simulink model "MARS1"  (R2022a)
settings: Solver=VariableStepAuto  StartTime=0.0  StopTime=inf  RelTol=1e-3
InitFcn:
  | links = gzlink("list","ingenuity");
  | for i=1:length(links)
  | gzlink("set","ingenuity",links(i),"Gravity","off");
  | end
model workspace (MAT data in the model file):
  T0 = -23.4
  h_trop = 7
  ingenuityParams : object (value not decoded)
values from neighbouring files (symbols this model uses):
  ingenuityParams =     [marsBatParam.mat]
undefined symbols (not defined in the file or in its folder): body, collective1, collective2, duration, ingenuity, leg1, leg2, leg3, leg4, link_name, model_name, rotor1, rotor2, solarPanel, world_pose
libraries: fl_lib x35, robotgazebolib x31, nesl_utility x12, ee_lib x11, slpidlib x7, simulink x4, sharedtransform x2, shared6dof x1, aerolibwind2 x1
(part 2 of 3)

== system MARS1/Gazebo Simulation/Link Body6 ==
  In1 : Inport
  In2 : Inport  Port=2
  In3 : Inport  Port=3
  In4 : Inport  Port=4
  In5 : Inport  Port=5
  In6 : Inport  Port=6
  In7 : Inport  Port=7
  In8 : Inport  Port=8
  Bus Assignment : BusAssignment  AssignedSignals=model_name,link_name,world_pose.position.x,world_pose.position.y,world_pose.position.z,world_pose.orientation.w,world_pose.orientation.x,world_pose.orientation.y,world_pose.orientation.z,duration.seconds
  Gazebo Blank Message : robotgazebolib/Gazebo Blank Message  msgType=SetLinkWorldPose  sampleTime=0.01  busName='Gazebo_SL_Bus_gazebo_msgs_SetLinkWorldPose'
      settings: SourceProductBaseCode=RO
  Gazebo Select Entity : robotgazebolib/Gazebo Select Entity  modelElemName=ingenuity/collective1  outputArraySize=128  OutputLabel=Link  SelectType=Link
      settings: SourceProductBaseCode=RO
  Out1 : Outport
  wires:
  In6/1 -> Bus Assignment/9
  In4/1 -> Bus Assignment/7
  In3/1 -> Bus Assignment/6
  In7/1 -> Bus Assignment/10
  In2/1 -> Bus Assignment/5
  Bus Assignment/1 -> Out1/1
  Gazebo Select Entity/2 -> Bus Assignment/3
  In5/1 -> Bus Assignment/8
  Gazebo Blank Message/1 -> Bus Assignment/1
  In8/1 -> Bus Assignment/11
  In1/1 -> Bus Assignment/4
  Gazebo Select Entity/1 -> Bus Assignment/2

== system MARS1/Gazebo Simulation/Link Body7 ==
  In1 : Inport
  In2 : Inport  Port=2
  In3 : Inport  Port=3
  In4 : Inport  Port=4
  In5 : Inport  Port=5
  In6 : Inport  Port=6
  In7 : Inport  Port=7
  In8 : Inport  Port=8
  Bus Assignment : BusAssignment  AssignedSignals=model_name,link_name,world_pose.position.x,world_pose.position.y,world_pose.position.z,world_pose.orientation.w,world_pose.orientation.x,world_pose.orientation.y,world_pose.orientation.z,duration.seconds
  Gazebo Blank Message : robotgazebolib/Gazebo Blank Message  msgType=SetLinkWorldPose  sampleTime=0.01  busName='Gazebo_SL_Bus_gazebo_msgs_SetLinkWorldPose'
      settings: SourceProductBaseCode=RO
  Gazebo Select Entity : robotgazebolib/Gazebo Select Entity  modelElemName=ingenuity/rotor1  outputArraySize=128  OutputLabel=Link  SelectType=Link
      settings: SourceProductBaseCode=RO
  Out1 : Outport
  wires:
  Gazebo Select Entity/1 -> Bus Assignment/2
  In1/1 -> Bus Assignment/4
  In8/1 -> Bus Assignment/11
  Gazebo Blank Message/1 -> Bus Assignment/1
  In5/1 -> Bus Assignment/8
  Gazebo Select Entity/2 -> Bus Assignment/3
  Bus Assignment/1 -> Out1/1
  In2/1 -> Bus Assignment/5
  In7/1 -> Bus Assignment/10
  In3/1 -> Bus Assignment/6
  In4/1 -> Bus Assignment/7
  In6/1 -> Bus Assignment/9

== system MARS1/Gazebo Simulation/Link Body8 ==
  In1 : Inport
  In2 : Inport  Port=2
  In3 : Inport  Port=3
  In4 : Inport  Port=4
  In5 : Inport  Port=5
  In6 : Inport  Port=6
  In7 : Inport  Port=7
  In8 : Inport  Port=8
  Bus Assignment : BusAssignment  AssignedSignals=model_name,link_name,world_pose.position.x,world_pose.position.y,world_pose.position.z,world_pose.orientation.w,world_pose.orientation.x,world_pose.orientation.y,world_pose.orientation.z,duration.seconds
  Gazebo Blank Message : robotgazebolib/Gazebo Blank Message  msgType=SetLinkWorldPose  sampleTime=0.01  busName='Gazebo_SL_Bus_gazebo_msgs_SetLinkWorldPose'
      settings: SourceProductBaseCode=RO
  Gazebo Select Entity : robotgazebolib/Gazebo Select Entity  modelElemName=ingenuity/body  outputArraySize=128  OutputLabel=Link  SelectType=Link
      settings: SourceProductBaseCode=RO
  Out1 : Outport
  wires:
  In6/1 -> Bus Assignment/9
  In4/1 -> Bus Assignment/7
  In3/1 -> Bus Assignment/6
  In7/1 -> Bus Assignment/10
  In2/1 -> Bus Assignment/5
  Bus Assignment/1 -> Out1/1
  Gazebo Select Entity/2 -> Bus Assignment/3
  In5/1 -> Bus Assignment/8
  Gazebo Blank Message/1 -> Bus Assignment/1
  In8/1 -> Bus Assignment/11
  In1/1 -> Bus Assignment/4
  Gazebo Select Entity/1 -> Bus Assignment/2

== system MARS1/Gazebo Simulation/Link Body9 ==
  In1 : Inport
  In2 : Inport  Port=2
  In3 : Inport  Port=3
  In4 : Inport  Port=4
  In5 : Inport  Port=5
  In6 : Inport  Port=6
  In7 : Inport  Port=7
  In8 : Inport  Port=8
  Bus Assignment : BusAssignment  AssignedSignals=model_name,link_name,world_pose.position.x,world_pose.position.y,world_pose.position.z,world_pose.orientation.w,world_pose.orientation.x,world_pose.orientation.y,world_pose.orientation.z,duration.seconds
  Gazebo Blank Message : robotgazebolib/Gazebo Blank Message  msgType=SetLinkWorldPose  sampleTime=0.01  busName='Gazebo_SL_Bus_gazebo_msgs_SetLinkWorldPose'
      settings: SourceProductBaseCode=RO
  Gazebo Select Entity : robotgazebolib/Gazebo Select Entity  modelElemName=ingenuity/leg4  outputArraySize=128  OutputLabel=Link  SelectType=Link
      settings: SourceProductBaseCode=RO
  Out1 : Outport
  wires:
  Gazebo Select Entity/1 -> Bus Assignment/2
  In1/1 -> Bus Assignment/4
  In8/1 -> Bus Assignment/11
  Gazebo Blank Message/1 -> Bus Assignment/1
  In5/1 -> Bus Assignment/8
  Gazebo Select Entity/2 -> Bus Assignment/3
  Bus Assignment/1 -> Out1/1
  In2/1 -> Bus Assignment/5
  In7/1 -> Bus Assignment/10
  In3/1 -> Bus Assignment/6
  In4/1 -> Bus Assignment/7
  In6/1 -> Bus Assignment/9

== system MARS1/Gazebo Simulation/Rot2Quat ==
  "R1, R2, R3" : Inport
  Demux : Demux
  Rate w : RateTransition
  Rate x : RateTransition
  Rate y : RateTransition
  Rate z : RateTransition
  Rotation Angles to Quaternions : sharedtransform/Rotation Angles to Quaternions  rotationOrder=XYZ  aMode=aMode
      settings: SourceProductBaseCode=AE,PW,DR,MT,VE
  Out1 : Outport
  Out2 : Outport  Port=2
  Out3 : Outport  Port=3
  Out4 : Outport  Port=4
  wires:
  Demux/3 -> Rate y/1
  Demux/2 -> Rate x/1
  Demux/1 -> Rate w/1
  Demux/4 -> Rate z/1
  Rate x/1 -> Out2/1
  Rotation Angles to Quaternions/1 -> Demux/1
  "R1, R2, R3"/1 -> Rotation Angles to Quaternions/1
  Rate y/1 -> Out3/1
  Rate w/1 -> Out1/1
  Rate z/1 -> Out4/1

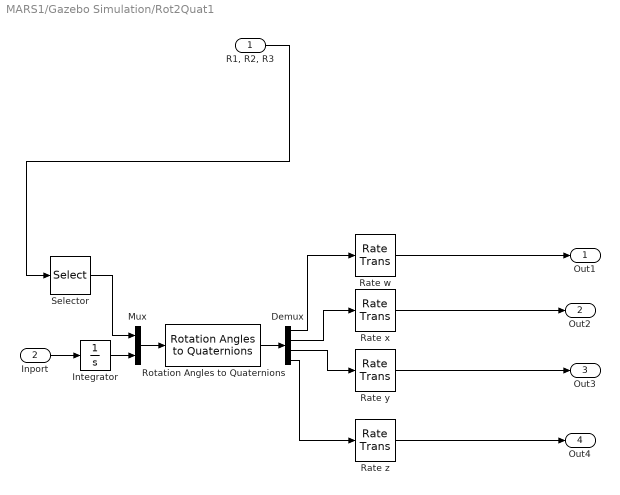
== system MARS1/Gazebo Simulation/Rot2Quat1 ==
  "R1, R2, R3" : Inport
  Inport : Inport  Port=2
  Demux : Demux
  Integrator : Integrator
  Mux : Mux  Inputs=2
  Rate w : RateTransition
  Rate x : RateTransition
  Rate y : RateTransition
  Rate z : RateTransition
  Rotation Angles to Quaternions : sharedtransform/Rotation Angles to Quaternions  rotationOrder=XYZ  aMode=aMode
      settings: SourceProductBaseCode=AE,PW,DR,MT,VE
  Selector : Selector  InputPortWidth=3  IndexOptions=Index vector (dialog)  Indices=[1 2]  OutputSizes=1
  Out1 : Outport
  Out2 : Outport  Port=2
  Out3 : Outport  Port=3
  Out4 : Outport  Port=4
  wires:
  Rate z/1 -> Out4/1
  Rate w/1 -> Out1/1
  Rate y/1 -> Out3/1
  Rotation Angles to Quaternions/1 -> Demux/1
  Rate x/1 -> Out2/1
  Demux/4 -> Rate z/1
  Demux/1 -> Rate w/1
  Demux/2 -> Rate x/1
  Demux/3 -> Rate y/1
  Mux/1 -> Rotation Angles to Quaternions/1
  Selector/1 -> Mux/1
  "R1, R2, R3"/1 -> Selector/1
  Integrator/1 -> Mux/2
  Inport/1 -> Integrator/1

== system MARS1/Gazebo Simulation/xyz ==
  In1 : Inport
  Demux1 : Demux  Outputs=3
  Rate Transition : RateTransition
  Rate Transition1 : RateTransition
  Rate Transition2 : RateTransition
  Out1 : Outport
  Out2 : Outport  Port=2
  Out3 : Outport  Port=3
  wires:
  Demux1/3 -> Rate Transition2/1
  Demux1/1 -> Rate Transition/1
  Demux1/2 -> Rate Transition1/1
  In1/1 -> Demux1/1
  Rate Transition/1 -> Out1/1
  Rate Transition1/1 -> Out2/1
  Rate Transition2/1 -> Out3/1

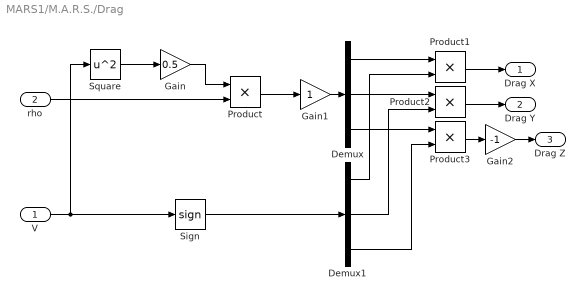
== system MARS1/M.A.R.S./Drag ==
  V : Inport
  rho : Inport  Port=2
  Demux : Demux  Outputs=3
  Demux1 : Demux  Outputs=3
  Gain : Gain  Gain=0.5
  Gain1 : Gain
  Gain2 : Gain  Gain=-1
  Product{,1..3} (4 alike) : Product
  Sign : Signum
  Square : Math  Operator=square
  Drag X : Outport
  Drag Y : Outport  Port=2
  Drag Z : Outport  Port=3
  wires:
  V/1 -> Square/1, Sign/1
  Demux1/3 -> Product3/2
  Demux1/2 -> Product2/2
  Demux/3 -> Product3/1
  Gain/1 -> Product/1
  Gain1/1 -> Demux/1
  rho/1 -> Product/2
  Square/1 -> Gain/1
  Demux1/1 -> Product1/2
  Product/1 -> Gain1/1
  Product1/1 -> Drag X/1
  Demux/1 -> Product1/1
  Demux/2 -> Product2/1
  Sign/1 -> Demux1/1
  Product2/1 -> Drag Y/1
  Product3/1 -> Gain2/1
  Gain2/1 -> Drag Z/1

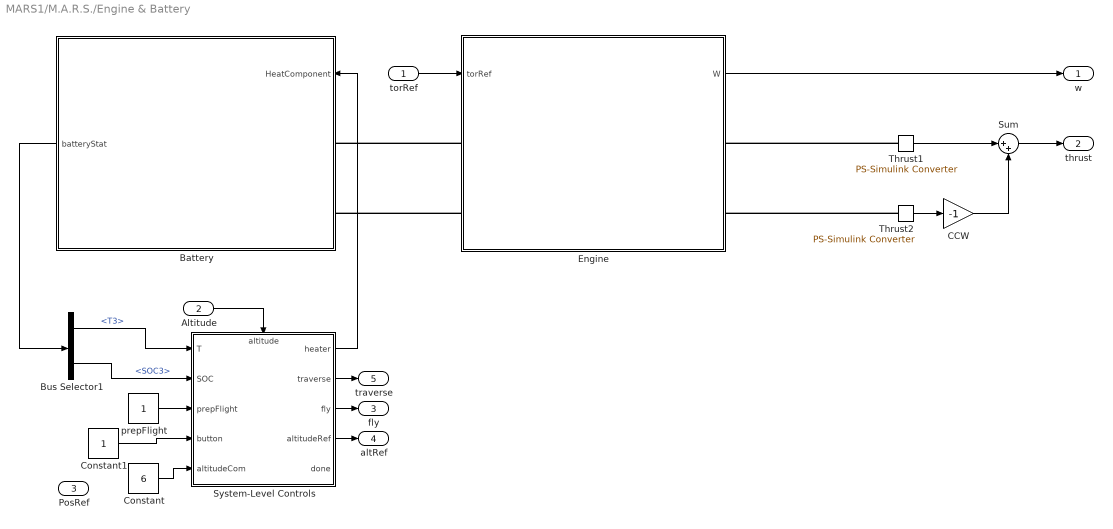
== system MARS1/M.A.R.S./Engine & Battery ==
  torRef : Inport
  Altitude : Inport  Port=2
  PosRef : Inport  Port=3
  Battery : Subsystem
      mask Display: image('$imagefile'); % Use "Edit Image" on toolstrip to change.
  Bus Selector1 : BusSelector  OutputSignals=T3,SOC3
  CCW : Gain  Gain=-1
  Constant : Constant  Value=6
  Constant1 : Constant
  Engine : Subsystem
      mask Display: image('$imagefile'); % Use "Edit Image" on toolstrip to change.
  Sum : Sum  Inputs=|++
  System-Level Controls : Stateflow chart  TreatAsAtomicUnit=on
      settings: PortSchema="{\"entries\":[{\"content\":{\"sides\":[{\"content\":{\"connectorIds\":[\"In2\",\"In3\",\"In5\",\"In4\",\"In1\"]},\"type\":\"ConnectorPlacement.EquallySpacedRectSide\",\"uuid\":\"5067341e-d12a-4a2a-9253-3fb06d0079cf\"},{\"content\":{\"connectorIds\":[\"Out1\",\"Out2\",\"Out3\",\"Out4\",\"Out5\"],\"side\":\"RIGHT\"},\"type\":\"ConnectorPlacement.EquallySpacedRectSide\",\"uuid\":\"5404e1d9-f923-45fb-998d-e24e5a5fd6b6\"},{\"content\":{\"connectorIds\":[\"In6\"],\"side\":\"TOP\"},\"type\":\"ConnectorPlacement.EquallySpacedRectSide\",\"uuid\":\"b72b8578-46c7-4b5e-a689-fe24a80a6d63\"}]},\"type\":\"ConnectorPlacement.EquallySpacedConnector\",\"uuid\":\"f5827d07-5d2a-4259-8e8b-6d4ada56c462\"}],\"packageUris\":[\"http://schema.mathworks.com/mf0/Connector/R2020b\"],\"version\":\"1.0\"}"
  Thrust1 : nesl_utility/PS-Simulink Converter  PhysicalDomain=network_engine_domain  SubClassName=ps_output  LeftPortType=input  RightPortType=output  PseudoPeriodic=off  Frequencies=[]  VectorFormat=inherit  Unit=inherit  AffineConversion=off
      settings: SourceProductBaseCode=SS,PW,VE
  Thrust2 : nesl_utility/PS-Simulink Converter  PhysicalDomain=network_engine_domain  SubClassName=ps_output  LeftPortType=input  RightPortType=output  PseudoPeriodic=off  Frequencies=[]  VectorFormat=inherit  Unit=inherit  AffineConversion=off
      settings: SourceProductBaseCode=SS,PW,VE
  prepFlight : Constant
  w : Outport
  thrust : Outport  Port=2
  fly : Outport  Port=3
  altRef : Outport  Port=4
  traverse : Outport  Port=5
  wires:
  Thrust2/1 -> CCW/1
  Sum/1 -> thrust/1
  System-Level Controls/1(heater) -> Battery/1(HeatComponent)
  Battery/1(batteryStat) -> Bus Selector1/1
  System-Level Controls/3(fly) -> fly/1
  Bus Selector1/2 -> System-Level Controls/3(SOC)  "<SOC3>"
  Bus Selector1/1 -> System-Level Controls/2(T)  "<T3>"
  System-Level Controls/4(altitudeRef) -> altRef/1
  prepFlight/1 -> System-Level Controls/5(prepFlight)
  Altitude/1 -> System-Level Controls/6(altitude)
  Constant/1 -> System-Level Controls/1(altitudeCom)
  Thrust1/1 -> Sum/1
  CCW/1 -> Sum/2
  torRef/1 -> Engine/1(torRef)
  Engine/1(W) -> w/1
  System-Level Controls/2(traverse) -> traverse/1
  Constant1/1 -> System-Level Controls/4(button)
  connections:
  Thrust1/LConn1 -- Engine/RConn1
  Engine/LConn1 -- Battery/LConn1
  Engine/LConn2 -- Battery/LConn2
  Thrust2/LConn1 -- Engine/RConn2

== system MARS1/M.A.R.S./Force Components ==
  note: Subsystem
  In1 : Inport
  In2 : Inport  Port=2
  delta : Inport  Port=3
  epsilon : Inport  Port=4
  Components : Subsystem
  Product2 : Product
  Subsystem : Subsystem
  Out1 : Outport
  Out2 : Outport  Port=2
  Out3 : Outport  Port=3
  wires:
  Components/2(Out2) -> Subsystem/3(In3)
  Components/1(Out1) -> Subsystem/2(In2)
  Components/3(Out3) -> Subsystem/4(In4)
  In1/1 -> Product2/1
  Components/4(Out4) -> Subsystem/5(In5)
  epsilon/1 -> Components/2(epsilon)
  Subsystem/1(Out1) -> Out1/1
  Product2/1 -> Subsystem/1(In1)
  delta/1 -> Components/1(delta)
  In2/1 -> Product2/2
  Subsystem/3(Out3) -> Out3/1
  Subsystem/2(Out2) -> Out2/1

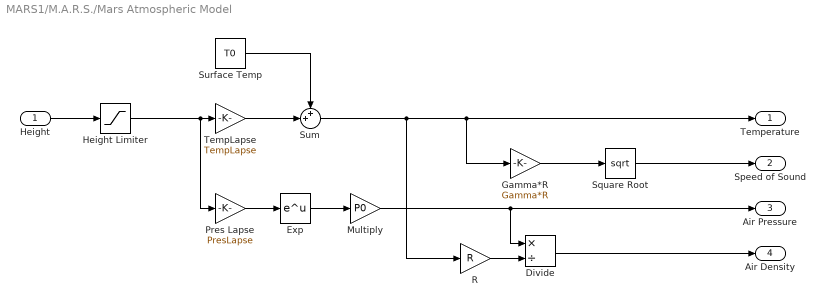
== system MARS1/M.A.R.S./Mars Atmospheric Model ==
  Height : Inport
  Divide : Product  Inputs=*/
  Exp : Math
  Gamma*R : Gain  Gain=Gamma*R
  Height Limiter : Saturate  UpperLimit=height_lim  LowerLimit=0
  Multiply : Gain  Gain=P0
  Pres Lapse : Gain  Gain=PresLapse
  R : Gain  Gain=R
  Square Root : Sqrt
  Sum : Sum  Inputs=++|
  Surface Temp : Constant  Value=T0
  TempLapse : Gain  Gain=TempLapse
  Temperature : Outport  Unit=K  VectorParamsAs1DForOutWhenUnconnected=off
  Speed of Sound : Outport  Port=2  Unit=m/s  VectorParamsAs1DForOutWhenUnconnected=off
  Air Pressure : Outport  Port=3  Unit=Pa  VectorParamsAs1DForOutWhenUnconnected=off
  Air Density : Outport  Port=4  Unit=kg/m^3  VectorParamsAs1DForOutWhenUnconnected=off
  wires:
  TempLapse/1 -> Sum/2
  Surface Temp/1 -> Sum/1
  Sum/1 -> Gamma*R/1, Temperature/1, R/1
  Pres Lapse/1 -> Exp/1
  Exp/1 -> Multiply/1
  Multiply/1 -> Divide/1, Air Pressure/1
  Height/1 -> Height Limiter/1
  Height Limiter/1 -> Pres Lapse/1, TempLapse/1
  Gamma*R/1 -> Square Root/1
  Square Root/1 -> Speed of Sound/1
  R/1 -> Divide/2
  Divide/1 -> Air Density/1

== system MARS1/Translate - Experimental/Distance Calc ==
  In1 : Inport
  In2 : Inport  Port=2
  Square : Math  Operator=square
  Square Root : Sqrt
  Square1 : Math  Operator=square
  Sum : Sum  Inputs=|++
  dist : Outport
  wires:
  Sum/1 -> Square Root/1
  Square Root/1 -> dist/1
  Square1/1 -> Sum/2
  Square/1 -> Sum/1
  In1/1 -> Square/1
  In2/1 -> Square1/1

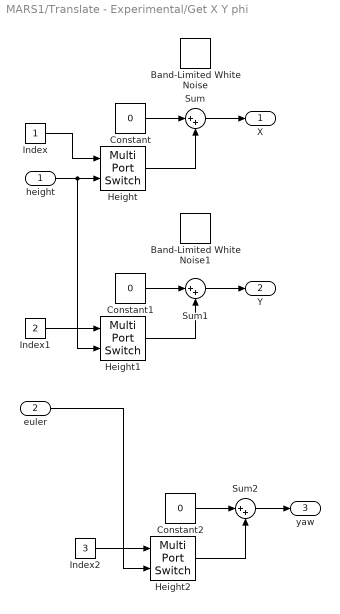
== system MARS1/Translate - Experimental/Get X Y phi ==
  height : Inport
  euler : Inport  Port=2
  Band-Limited White Noise : simulink/Sources/Band-Limited White Noise  Cov=[0.1]  Ts=0.1  seed=[23341]
  Band-Limited White Noise1 : simulink/Sources/Band-Limited White Noise  Cov=[0.1]  Ts=0.1  seed=[23341]
  Constant : Constant  Value=0
  Constant1 : Constant  Value=0
  Constant2 : Constant  Value=0
  Height : MultiPortSwitch  Inputs=1  SaturateOnIntegerOverflow=off  InputSameDT=off
  Height1 : MultiPortSwitch  Inputs=1  SaturateOnIntegerOverflow=off  InputSameDT=off
  Height2 : MultiPortSwitch  Inputs=1  SaturateOnIntegerOverflow=off  InputSameDT=off
  Index : Constant
  Index1 : Constant  Value=2
  Index2 : Constant  Value=3
  Sum : Sum  Inputs=|++
  Sum1 : Sum  Inputs=|++
  Sum2 : Sum  Inputs=|++
  X : Outport
  Y : Outport  Port=2
  yaw : Outport  Port=3
  wires:
  Constant/1 -> Sum/1
  Height/1 -> Sum/2
  Index1/1 -> Height1/1
  Height1/1 -> Sum1/2
  Index/1 -> Height/1
  Sum1/1 -> Y/1
  height/1 -> Height/2, Height1/2
  Sum/1 -> X/1
  Constant1/1 -> Sum1/1
  Constant2/1 -> Sum2/1
  euler/1 -> Height2/2
  Sum2/1 -> yaw/1
  Height2/1 -> Sum2/2
  Index2/1 -> Height2/1

== system MARS1/Translate - Experimental/Position Hold ==
  dx : Inport
  dy : Inport  Port=2
  yaw : Inport  Port=3
  dist : Inport  Port=4
  " PID Controller" : slpidlib/PID Controller  Controller=PID  Form=Parallel  TimeDomain=Continuous-time  UseExternalTs=off  SampleTime=-1  IntegratorMethod=Forward Euler  FilterMethod=Forward Euler  ControllerParametersSource=internal  P=2.75291380025279  I=0.654733901603954  UseKiTs=off  D=2.09643844624086  N=374.082600822232  UseFilter=on  TunerSelectOption=Transfer Function Based (PID Tuner App)  ZeroCross=off  InitialConditionSource=internal  InitialConditionForIntegrator=0  InitialConditionForFilter=0  DifferentiatorICPrevScaledInput=0  ExternalReset=none  TrackingMode=off  Kt=1  LimitOutput=on  SatLimitsSource=internal  UpperSaturationLimit=3  LowerSaturationLimit=-3  LinearizeAsGain=off  AntiWindupMode=clamping  Kb=1  POutMin=[]  POutMax=[]  IOutMin=[]  IOutMax=[]  DOutMin=[]  DOutMax=[]  NOutMin=[]  NOutMax=[]  SumOutMin=[]  SumOutMax=[]  SaturationOutMin=[]  SaturationOutMax=[]  PParamMin=[]  PParamMax=[]  IParamMin=[]  IParamMax=[]  DParamMin=[]  DParamMax=[]  NParamMin=[]  NParamMax=[]  KbParamMin=[]  KbParamMax=[]  KtParamMin=[]  KtParamMax=[]  KbOutMin=[]  KbOutMax=[]  KtOutMin=[]  KtOutMax=[]  IntegratorOutMin=[]  IntegratorOutMax=[]  FilterOutMin=[]  FilterOutMax=[]  SumI1OutMin=[]  SumI1OutMax=[]  SumI2OutMin=[]  SumI2OutMax=[]  SumI3OutMin=[]  SumI3OutMax=[]  SumI4OutMin=[]  SumI4OutMax=[]  SumDOutMin=[]  SumDOutMax=[]  DifferentiatorOutMin=[]  DifferentiatorOutMax=[]  FilterDiffOutCoefMin=[]  FilterDiffOutCoefMax=[]  ReciprocalOutMin=[]  ReciprocalOutMax=[]  SumDenOutMin=[]  SumDenOutMax=[]  SumNumOutMin=[]  SumNumOutMax=[]  DivideOutMin=[]  DivideOutMax=[]  UdiffTsProdOutMin=[]  UdiffTsProdOutMax=[]  NTsProdOutMin=[]  NTsProdOutMax=[]  UintegralTsProdOutMin=[]  UintegralTsProdOutMax=[]  UngainTsProdOutMin=[]  UngainTsProdOutMax=[]  IntegratorContinuousStateAttributes=''  IntegratorStateMustResolveToSignalObject=off  IntegratorRTWStateStorageClass=Auto  FilterContinuousStateAttributes=''  FilterStateMustResolveToSignalObject=off  FilterRTWStateStorageClass=Auto  ParallelPVariant=InternalParameters  IdealPVariant=Disabled  IVariant=InternalParameters  DVariant=InternalParameters  IntegratorVariant=Continuous  SatVariant=Enabled  AWVariant=ContClampingParallel  PCopyVariant=Disabled  TRVariant=Disabled  FdbkBlocksVariant=Forward  IdealPFdbkVariant=Disabled  SatFdbkVariant=Disabled  DerivativeFilterVariant=ContFilter  NVariant=InternalParameters  NCopyVariant=Disabled  FilterICVariant=InternalICsFilter  IntegratorICVariant=InternalICs  ExternalResetVariant=Disabled  TRSumVariant=Passthrough  SumFdbkVariant=Disabled  SumVariant=Sum_PID  TsampFilterVariant=InternalTs  TsampNgainVariant=Passthrough  TsampIntegralVariant=Passthrough  ExternalSaturationOutDataTypeStr=Inherit: Same as second input  aMode=0
  Add1 : Sum  Inputs=+-
  Add3 : Sum  Inputs=+-
  Derivative : TransferFcn  Numerator=[1 0]  Denominator=[1e-1 1]
  Distance Calc : Subsystem
  Tan : Trigonometry  Operator=atan2
  Velocity PID Controller : slpidlib/PID Controller  Controller=PID  Form=Parallel  TimeDomain=Continuous-time  UseExternalTs=off  SampleTime=-1  IntegratorMethod=Forward Euler  FilterMethod=Forward Euler  ControllerParametersSource=internal  P=155.19306060889  I=41.1553609138668  UseKiTs=off  D=46.7041807942439  N=1.30346385486406  UseFilter=on  TunerSelectOption=Transfer Function Based (PID Tuner App)  ZeroCross=off  InitialConditionSource=internal  InitialConditionForIntegrator=0  InitialConditionForFilter=0  DifferentiatorICPrevScaledInput=0  ExternalReset=none  TrackingMode=off  Kt=1  LimitOutput=on  SatLimitsSource=internal  UpperSaturationLimit=0.4  LowerSaturationLimit=-0.4  LinearizeAsGain=off  AntiWindupMode=clamping  Kb=1  POutMin=[]  POutMax=[]  IOutMin=[]  IOutMax=[]  DOutMin=[]  DOutMax=[]  NOutMin=[]  NOutMax=[]  SumOutMin=[]  SumOutMax=[]  SaturationOutMin=[]  SaturationOutMax=[]  PParamMin=[]  PParamMax=[]  IParamMin=[]  IParamMax=[]  DParamMin=[]  DParamMax=[]  NParamMin=[]  NParamMax=[]  KbParamMin=[]  KbParamMax=[]  KtParamMin=[]  KtParamMax=[]  KbOutMin=[]  KbOutMax=[]  KtOutMin=[]  KtOutMax=[]  IntegratorOutMin=[]  IntegratorOutMax=[]  FilterOutMin=[]  FilterOutMax=[]  SumI1OutMin=[]  SumI1OutMax=[]  SumI2OutMin=[]  SumI2OutMax=[]  SumI3OutMin=[]  SumI3OutMax=[]  SumI4OutMin=[]  SumI4OutMax=[]  SumDOutMin=[]  SumDOutMax=[]  DifferentiatorOutMin=[]  DifferentiatorOutMax=[]  FilterDiffOutCoefMin=[]  FilterDiffOutCoefMax=[]  ReciprocalOutMin=[]  ReciprocalOutMax=[]  SumDenOutMin=[]  SumDenOutMax=[]  SumNumOutMin=[]  SumNumOutMax=[]  DivideOutMin=[]  DivideOutMax=[]  UdiffTsProdOutMin=[]  UdiffTsProdOutMax=[]  NTsProdOutMin=[]  NTsProdOutMax=[]  UintegralTsProdOutMin=[]  UintegralTsProdOutMax=[]  UngainTsProdOutMin=[]  UngainTsProdOutMax=[]  IntegratorContinuousStateAttributes=''  IntegratorStateMustResolveToSignalObject=off  IntegratorRTWStateStorageClass=Auto  FilterContinuousStateAttributes=''  FilterStateMustResolveToSignalObject=off  FilterRTWStateStorageClass=Auto  ParallelPVariant=InternalParameters  IdealPVariant=Disabled  IVariant=InternalParameters  DVariant=InternalParameters  IntegratorVariant=Continuous  SatVariant=Enabled  AWVariant=ContClampingParallel  PCopyVariant=Disabled  TRVariant=Disabled  FdbkBlocksVariant=Forward  IdealPFdbkVariant=Disabled  SatFdbkVariant=Disabled  DerivativeFilterVariant=ContFilter  NVariant=InternalParameters  NCopyVariant=Disabled  FilterICVariant=InternalICsFilter  IntegratorICVariant=InternalICs  ExternalResetVariant=Disabled  TRSumVariant=Passthrough  SumFdbkVariant=Disabled  SumVariant=Sum_PID  TsampFilterVariant=InternalTs  TsampNgainVariant=Passthrough  TsampIntegralVariant=Passthrough  ExternalSaturationOutDataTypeStr=Inherit: Same as second input  aMode=0
  delta : Outport  OutputWhenDisabled=reset  InitialOutput=0
  epsilon : Outport  Port=2
  wires:
  dx/1 -> Distance Calc/2(In2), Tan/2
  yaw/1 -> Add3/2
  Derivative/1 -> Add1/2
  dy/1 -> Distance Calc/1(In1), Tan/1
  Add1/1 -> Velocity PID Controller/1
  Add3/1 -> epsilon/1
  Tan/1 -> Add3/1
  " PID Controller"/1 -> Add1/1  "velRef"
  dist/1 -> Derivative/1
  Velocity PID Controller/1 -> delta/1  "deltaRef"
  Distance Calc/1(Out1) -> " PID Controller"/1

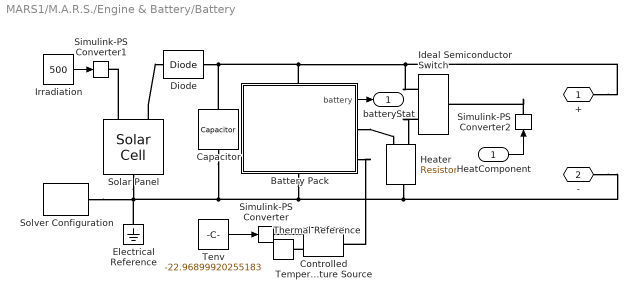
== system MARS1/M.A.R.S./Engine & Battery/Battery ==
  HeatComponent : Inport
  Battery Pack : Subsystem  Variant=on  VariantControlMode=label  LabelModeActiveChoice=Detailed Battery Pack
      settings: PortSchema="{\"entries\":[{\"content\":{\"sides\":[{\"content\":{\"connectorIds\":[]},\"type\":\"ConnectorPlacement.EquallySpacedRectSide\",\"uuid\":\"b9ff85f5-5d37-4551-b274-b4f400e31e90\"},{\"content\":{\"connectorIds\":[\"Out1\",\"RConn1\",\"RConn2\"],\"side\":\"RIGHT\"},\"type\":\"ConnectorPlacement.EquallySpacedRectSide\",\"uuid\":\"9895ebaf-077a-447d-9f12-67b2d221f552\"},{\"content\":{\"connectorIds\":[\"LConn1\"],\"side\":\"TOP\"},\"type\":\"ConnectorPlacement.EquallySpacedRectSide\",\"uuid\":\"1c6b4d28-0fee-40d3-aeb3-8529f8417079\"},{\"content\":{\"connectorIds\":[\"RConn3\"],\"side\":\"BOTTOM\"},\"type\":\"ConnectorPlacement.EquallySpacedRectSide\",\"uuid\":\"bb08ee4d-4e3f-4517-9dbc-020c674c7490\"}]},\"type\":\"ConnectorPlacement.EquallySpacedConnector\",\"uuid\":\"d782096a-eb61-452d-945f-a15e6ccd7694\"}],\"packageUris\":[\"http://schema.mathworks.com/mf0/Connector/R2020b\"],\"version\":\"1.0\"}"
  Capacitor : fl_lib/Electrical/Electrical Elements/Capacitor  c=1e-6 F  r=1e-3 Ohm  g=0 1/Ohm  i_specify=off  i_priority=None  i=0 A  i_nominal_specify=off  i_nominal_unit=A  i_nominal_value=1  v_specify=off  v_priority=None  v=0 V  v_nominal_specify=off  v_nominal_unit=V  v_nominal_value=1  vc_specify=on  vc_priority=High  vc=24 V  vc_nominal_specify=off  vc_nominal_unit=V  vc_nominal_value=1
      settings: SourceProductBaseCode=PW,SS,VE  LogSimulationData=on
  Controlled Temperature Source : fl_lib/Thermal/Thermal Sources/Controlled Temperature Source
      settings: SourceProductBaseCode=PW,SS,VE
  Diode : fl_lib/Electrical/Electrical Elements/Diode  Vf=0.6 V  Ron=0.3 Ohm  Goff=1e-8 1/Ohm  i_specify=off  i_priority=None  i=0 A  i_nominal_specify=off  i_nominal_unit=A  i_nominal_value=1  v_specify=off  v_priority=None  v=0 V  v_nominal_specify=off  v_nominal_unit=V  v_nominal_value=1
      settings: SourceProductBaseCode=PW,SS,VE  LogSimulationData=on
  Electrical Reference : fl_lib/Electrical/Electrical Elements/Electrical Reference
      settings: SourceProductBaseCode=PW,SS,VE
  Heater : ee_lib/Passive/Resistor  R=2 Ohm  enable_R_tol=0  R_tol=5  tol_distribution=1  nSigma=4  enable_operating_limits=0  operating_limit_action=2  max_working_voltage=100 V  power_rating=1 W  enable_faults=0  fault_action=1  R_faulted=inf Ohm  enable_temporal_fault=0  t_fault=1 s  enable_behavioral_fault=0  max_permissible_current=1 A  t_fail_on_current=1 s  noise_mode=0  sample_time=1e-3 s  repeatability=1  auto_seed=3499211588  user_seed=0  Tdevice=25 degC  power_derating_T1=70 degC  power_derating_T2=155 degC  operating_temperature_range_vec=[-50, 150] degC  alpha=3.93e-3 1/K  Tmeas=25 degC  thermal_mass=ingenuityParams.heater.thermalMass J/K  temperature_specify=on  temperature_priority=None  temperature=ingenuityParams.battery.cell.T_init degC  temperature_nominal_specify=off  temperature_nominal_unit=K  temperature_nominal_value=1
      settings: LogSimulationData=on  InternalSimscapePortConfiguration="{\"Bottom\":[],\"Left\":[{\"id\":\"p\",\"label\":\"+\",\"type\":\"foundation.electrical.electrical\"},{\"id\":\"H\",\"label\":\"H\",\"type\":\"foundation.thermal.thermal\"}],\"Right\":[{\"id\":\"n\",\"label\":\"-\",\"type\":\"foundation.electrical.electrical\"}],\"Top\":[]}"
  Ideal Semiconductor Switch : ee_lib/Semiconductors & Converters/Ideal Semiconductor Switch  Ron=0.001 Ohm  Goff=1e-6 1/Ohm  Vth=0.5 V  diode_param=1  diode_Vf=0.8 V  diode_Ron=0.001 Ohm  diode_Goff=1e-5 1/Ohm  diode_C=50e-9 F  diode_iRM=-235 A  diode_iF=300 A  diode_idot=-50 A/us  diode_trr_param=1  diode_trr_factor=3  diode_trr=15 us  diode_Qrr=1500 s*uA
      settings: SourceProductBaseCode=PS  LogSimulationData=on
  Irradiation : Constant  Value=500
  Simulink-PS Converter : nesl_utility/Simulink-PS Converter  PhysicalDomain=network_engine_domain  SubClassName=ps_input  LeftPortType=input  RightPortType=output  PseudoPeriodic=off  Frequencies=[]  NoiseDistribution=none  NoiseParameters=[]  Unit=degC  AffineConversion=on  FilteringAndDerivatives=provide  SimscapeFilterOrder=1  InputFilterTimeConstant=0.001  UdotUserProvided=0
      settings: SourceProductBaseCode=SS,PW,VE
  Simulink-PS Converter1 : nesl_utility/Simulink-PS Converter  PhysicalDomain=network_engine_domain  SubClassName=ps_input  LeftPortType=input  RightPortType=output  PseudoPeriodic=off  Frequencies=[]  NoiseDistribution=none  NoiseParameters=[]  Unit=W/m^2  AffineConversion=off  FilteringAndDerivatives=provide  SimscapeFilterOrder=1  InputFilterTimeConstant=0.001  UdotUserProvided=0
      settings: SourceProductBaseCode=SS,PW,VE
  Simulink-PS Converter2 : nesl_utility/Simulink-PS Converter  PhysicalDomain=network_engine_domain  SubClassName=ps_input  LeftPortType=input  RightPortType=output  PseudoPeriodic=off  Frequencies=[]  NoiseDistribution=none  NoiseParameters=[]  Unit=V  AffineConversion=off  FilteringAndDerivatives=provide  SimscapeFilterOrder=1  InputFilterTimeConstant=0.001  UdotUserProvided=0
      settings: SourceProductBaseCode=SS,PW,VE
  Solar Panel : ee_lib/Sources/Solar Cell  prm=1  Isc=ingenuityParams.solarcells.Isc A  Voc=ingenuityParams.solarcells.Voc V  Is=1e-6 A  Is2=0 A  Iph=7.34 A  Ir0=ingenuityParams.solarcells.Ir0 W/m^2  ec=ingenuityParams.solarcells.qualFactor  N2=2  Rs=ingenuityParams.solarcells.Rs Ohm  Rp=inf Ohm  N_series=ingenuityParams.solarcells.Nseries  N_parallel=ingenuityParams.solarcells.Nparallel  TIPH1=0 1/K  EG=1.11 eV  TXIS1=3  TXIS2=3  TRS1=0  TRP1=0  Tmeas=25 degC  TFIXED=25 degC  thermal_mass=100 J/K  initial_temperature=25 degC
      settings: SourceProductBaseCode=PS  LogSimulationData=on
  Solver Configuration : nesl_utility/Solver Configuration  PhysicalDomain=network_engine_domain  SubClassName=solver  LeftPortType=input  RightPortType=generic  Tones=[]  Harmonics=[]  SimulateNoise=off  Profile=off  UseLocalSampling=off  EnableSwitchedLinearOptims=on  FrequencyDomain=off  UseCCode=off  RelTol=0.001  AbsTol=1e-06  MinStep=1e-09  ToWorkspace=off  RevertToSquareIcSolve=off  NumHomotopyIterations=100  PhasorMode=off  PhasorModeNumHarmonics=1  IndexReductionMethod=DerivativeReplacement  DoDC=off  ResidualTolerance=1e-09  UseLocalSolver=off  LocalSolverChoice=NE_BACKWARD_EULER_ADVANCER  LocalSolverSampleTime=0.001  DoFixedCost=off  MaxNonlinIter=3  MaxModeIter=2  ComputeImpulses=off  ImpulseIterations=2  LinearAlgebra=auto  LinearAlgebraNumThread=0  EquationFormulation=NE_TIME_EF  DelaysMemoryBudget=1024  AutomaticFiltering=on  FilteringTimeConstant=0.001  PartitionStorageMethod=AS_NEEDED  PartitionMemoryBudget=1024  PartitionMethod=ROBUST
      settings: SourceProductBaseCode=SS,PW,VE
  Tenv : Constant  Value=-22.96899920255183
  Thermal Reference : fl_lib/Thermal/Thermal Elements/Thermal Reference
      settings: SourceProductBaseCode=PW,SS,VE
  + : PMIOPort  Side=Left
  - : PMIOPort  Port=2  Side=Left
  batteryStat : Outport
  wires:
  Tenv/1 -> Simulink-PS Converter/1
  Battery Pack/1(battery) -> batteryStat/1
  HeatComponent/1 -> Simulink-PS Converter2/1
  Irradiation/1 -> Simulink-PS Converter1/1
  connections:
  Solar Panel/LConn2 -- Diode/LConn1
  Capacitor/LConn1 -- +/RConn1 -- Ideal Semiconductor Switch/RConn1 -- Battery Pack/LConn1 -- Diode/RConn1
  Controlled Temperature Source/RConn1 -- Simulink-PS Converter/RConn1
  Heater/RConn1 -- -/RConn1 -- Solver Configuration/RConn1 -- Electrical Reference/LConn1 -- Solar Panel/RConn1 -- Capacitor/RConn1 -- Battery Pack/RConn3
  Simulink-PS Converter2/RConn1 -- Ideal Semiconductor Switch/LConn1
  Ideal Semiconductor Switch/RConn2 -- Heater/LConn1
  Controlled Temperature Source/RConn2 -- Thermal Reference/LConn1
  Solar Panel/LConn1 -- Simulink-PS Converter1/RConn1
  Battery Pack/RConn2 -- Controlled Temperature Source/LConn1
  Battery Pack/RConn1 -- Heater/LConn2

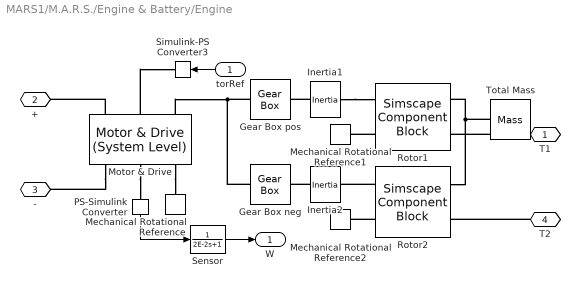
== system MARS1/M.A.R.S./Engine & Battery/Engine ==
  torRef : Inport
  Gear Box neg : fl_lib/Mechanical/Mechanisms/Gear Box  ratio=-1*ingenuityParams.gearbox.ratio  t_in_specify=off  t_in_priority=None  t_in=0 N*m  t_in_nominal_specify=off  t_in_nominal_unit=N*m  t_in_nominal_value=1  t_out_specify=off  t_out_priority=None  t_out=0 N*m  t_out_nominal_specify=off  t_out_nominal_unit=N*m  t_out_nominal_value=1
      settings: SourceProductBaseCode=PW,SS,VE  LogSimulationData=on
  Gear Box pos : fl_lib/Mechanical/Mechanisms/Gear Box  ratio=ingenuityParams.gearbox.ratio  t_in_specify=off  t_in_priority=None  t_in=0 N*m  t_in_nominal_specify=off  t_in_nominal_unit=N*m  t_in_nominal_value=1  t_out_specify=off  t_out_priority=None  t_out=0 N*m  t_out_nominal_specify=off  t_out_nominal_unit=N*m  t_out_nominal_value=1
      settings: SourceProductBaseCode=PW,SS,VE  LogSimulationData=on
  Inertia1 : fl_lib/Mechanical/Rotational Elements/Inertia  inertia=ingenuityParams.propeller.inertia kg*m^2  num_ports=foundation.enum.numPorts2.two  w_specify=off  w_priority=High  w=0 rad/s  w_nominal_specify=off  w_nominal_unit=rad/s  w_nominal_value=1  t_specify=off  t_priority=None  t=0 N*m  t_nominal_specify=off  t_nominal_unit=N*m  t_nominal_value=1
      settings: SourceProductBaseCode=PW,SS,VE  LogSimulationData=on  InternalSimscapePortConfiguration="{\"Bottom\":[],\"Left\":[{\"id\":\"I\",\"label\":\"\",\"type\":\"foundation.mechanical.rotational.rotational\"}],\"Right\":[{\"id\":\"J\",\"label\":\"\",\"type\":\"foundation.mechanical.rotational.rotational\"}],\"Top\":[]}"
  Inertia2 : fl_lib/Mechanical/Rotational Elements/Inertia  inertia=ingenuityParams.propeller.inertia kg*m^2  num_ports=foundation.enum.numPorts2.two  w_specify=off  w_priority=High  w=0 rad/s  w_nominal_specify=off  w_nominal_unit=rad/s  w_nominal_value=1  t_specify=off  t_priority=None  t=0 N*m  t_nominal_specify=off  t_nominal_unit=N*m  t_nominal_value=1
      settings: SourceProductBaseCode=PW,SS,VE  LogSimulationData=on  InternalSimscapePortConfiguration="{\"Bottom\":[],\"Left\":[{\"id\":\"I\",\"label\":\"\",\"type\":\"foundation.mechanical.rotational.rotational\"}],\"Right\":[{\"id\":\"J\",\"label\":\"\",\"type\":\"foundation.mechanical.rotational.rotational\"}],\"Top\":[]}"
  Mechanical Rotational Reference : fl_lib/Mechanical/Rotational Elements/Mechanical Rotational Reference
      settings: SourceProductBaseCode=PW,SS,VE
  Mechanical Rotational Reference1 : fl_lib/Mechanical/Rotational Elements/Mechanical Rotational Reference
      settings: SourceProductBaseCode=PW,SS,VE
  Mechanical Rotational Reference2 : fl_lib/Mechanical/Rotational Elements/Mechanical Rotational Reference
      settings: SourceProductBaseCode=PW,SS,VE
  Motor & Drive : ee_lib/Electromechanical/Motor & Drive (System Level)  torque_speed_param=ee.enum.electromech.envelope.torque_power  overtorque_param=ee.enum.electromech.overtorque.no  T_t=[.09, .08, .07, 0] N*m  T_t_intermittent=[.36, .32, .28, 0] N*m  T_t_2D=[.09, .09, .09; .08, .08, .08; .07, .07, .07; 0, 0, 0] N*m  T_t_intermittent_2D=[.36, .36, .36; .32, .32, .32; .28, .28, .28; 0, 0, 0] N*m  w_t=[0, 3750, 7500, 8000] rpm  vdc_t=[6, 12, 24] V  torque_max=ingenuityParams.motordrive.torMax N*m  power_max=ingenuityParams.motordrive.powMax W  torque_max_intermittent=0.4 N*m  power_max_intermittent=120 W  time_overtorque=30 s  time_recover=60 s  Tc=ingenuityParams.motordrive.Tc s  losses_param=1  eff=ingenuityParams.motordrive.effRated  w_eff=ingenuityParams.motordrive.wRated rpm  T_eff=ingenuityParams.motordrive.torRated N*m  Piron=ingenuityParams.motordrive.ironLoss W  Pbase=ingenuityParams.motordrive.fixedLoss W  w_eff_vec=[-8000, -4000, 0, 4000, 8000] rpm  T_eff_vec=[0, .03, .06, .09] N*m  v_eff_vec=[100, 250, 400] V  losses_mat=[1.49, 1.67, 2.21, 3.1; .42, .69, 1.14, 2.03; .06, .24, .78, 1.68; .42, .69, 1.14, 2.03; 1.49, 1.67, 2.21, 3.1] W  efficiency_mat=[95, 95, 95, 95; 95, 95, 95, 95; 95, 95, 95, 95; 95, 95, 95, 95; 95, 95, 95, 95]  losses_mat_3D=ones(5, 4, 3) W  efficiency_mat_3D=95 * ones(5, 4, 3)  Res=ingenuityParams.motordrive.supplyRes Ohm  enable_fault=simscape.enum.onoff.off  fault_condition=1  fault_threshold=0.5  J=0 kg*m^2  lam=0 N*m/(rad/s)  speed0=0 rpm  faulted_specify=off  faulted_priority=None  faulted=0  faulted_nominal_specify=off  faulted_nominal_unit=1  faulted_nominal_value=1  torqueLimitContinuous_specify=off  torqueLimitContinuous_priority=None  torqueLimitContinuous=0 N*m  torqueLimitContinuous_nominal_specify=off  torqueLimitContinuous_nominal_unit=N*m  torqueLimitContinuous_nominal_value=1  alpha=3.93e-3 1/K  Tmeas=25 degC  Tmeas2=125 degC  losses_mat_T2=[1.49, 1.74, 2.49, 3.74; .42, .67, 1.42, 2.67; .06, .31, 1.06, 2.31; .42, .67, 1.42, 2.67; 1.49, 1.74, 2.49, 3.74] W  efficiency_mat_T2=[95, 95, 95, 95; 95, 95, 95, 95; 95, 95, 95, 95; 95, 95, 95, 95; 95, 95, 95, 95]  losses_mat_3D_T2=ones(5, 4, 3) W  efficiency_mat_3D_T2=95 * ones(5, 4, 3)  thermal_mass=100 J/K  initial_temperature=25 degC
      settings: SourceProductBaseCode=PS  LogSimulationData=on
  PS-Simulink Converter : nesl_utility/PS-Simulink Converter  PhysicalDomain=network_engine_domain  SubClassName=ps_output  LeftPortType=input  RightPortType=output  PseudoPeriodic=off  Frequencies=[]  VectorFormat=1-D array  Unit=rad/s  AffineConversion=off
      settings: SourceProductBaseCode=SS,PW,VE
  Rotor1 : SimscapeComponentBlock  SourceFile=simple_rotor  ComponentPath=simple_rotor  ComponentVariants="[\"simple_rotor\"]"  ComponentVariantNames="[\"simple_rotor\"]"  ClassName=simple_rotor  SchemaVersion=1  rot_dir=simscape.enum.posneg.positive  D=ingenuityParams.propeller.diameter m  J_TLU=ingenuityParams.propeller.Jvec  k_thrust_TLU=ingenuityParams.propeller.kTvec  k_power_TLU=ingenuityParams.propeller.kPvec  interp_method=simscape.enum.interpolation.smooth  extrap_method=simscape.enum.extrapolation.linear  density=ingenuityParams.environment.atmDensity kg/m^3  n_thr=1e-2 Hz  w_specify=on  w_priority=None  w=0 rpm  w_nominal_specify=off  w_nominal_unit=rad/s  w_nominal_value=1  Q_specify=off  Q_priority=None  Q=0 N*m  Q_nominal_specify=off  Q_nominal_unit=N*m  Q_nominal_value=1
      settings: CopyFcn=simscape.engine.sli.internal.componentblockcallback(gcbh,'COPY')  PreCopyFcn=simscape.engine.sli.internal.componentblockcallback(gcbh,'PRECOPY')  PreDeleteFcn=simscape.engine.sli.internal.componentblockcallback(gcbh,'PREDELETE')  InternalSimscapePortConfiguration="{\"Bottom\":[],\"Left\":[{\"id\":\"R\",\"label\":\"R\",\"type\":\"foundation.mechanical.rotational.rotational\"},{\"id\":\"C\",\"label\":\"C\",\"type\":\"foundation.mechanical.rotational.rotational\"}],\"Right\":[{\"id\":\"V\",\"label\":\"V\",\"type\":\"foundation.mechanical.translational.translational\"},{\"id\":\"T\",\"label\":\"T\",\"type\":\"output\"}],\"Top\":[]}"
      mask Type: Simple Rotor
  Rotor2 : SimscapeComponentBlock  SourceFile=simple_rotor  ComponentPath=simple_rotor  ComponentVariants="[\"simple_rotor\"]"  ComponentVariantNames="[\"simple_rotor\"]"  ClassName=simple_rotor  SchemaVersion=1  rot_dir=simscape.enum.posneg.positive  D=ingenuityParams.propeller.diameter m  J_TLU=ingenuityParams.propeller.Jvec  k_thrust_TLU=ingenuityParams.propeller.kTvec  k_power_TLU=ingenuityParams.propeller.kPvec  interp_method=simscape.enum.interpolation.smooth  extrap_method=simscape.enum.extrapolation.linear  density=ingenuityParams.environment.atmDensity kg/m^3  n_thr=1e-2 Hz  w_specify=on  w_priority=None  w=0 rpm  w_nominal_specify=off  w_nominal_unit=rad/s  w_nominal_value=1  Q_specify=off  Q_priority=None  Q=0 N*m  Q_nominal_specify=off  Q_nominal_unit=N*m  Q_nominal_value=1
      settings: CopyFcn=simscape.engine.sli.internal.componentblockcallback(gcbh,'COPY')  PreCopyFcn=simscape.engine.sli.internal.componentblockcallback(gcbh,'PRECOPY')  PreDeleteFcn=simscape.engine.sli.internal.componentblockcallback(gcbh,'PREDELETE')  InternalSimscapePortConfiguration="{\"Bottom\":[],\"Left\":[{\"id\":\"R\",\"label\":\"R\",\"type\":\"foundation.mechanical.rotational.rotational\"},{\"id\":\"C\",\"label\":\"C\",\"type\":\"foundation.mechanical.rotational.rotational\"}],\"Right\":[{\"id\":\"V\",\"label\":\"V\",\"type\":\"foundation.mechanical.translational.translational\"},{\"id\":\"T\",\"label\":\"T\",\"type\":\"output\"}],\"Top\":[]}"
      mask Type: Simple Rotor
  Sensor : TransferFcn  Denominator=[2E-2 1]
  Simulink-PS Converter3 : nesl_utility/Simulink-PS Converter  PhysicalDomain=network_engine_domain  SubClassName=ps_input  LeftPortType=input  RightPortType=output  PseudoPeriodic=off  Frequencies=[]  NoiseDistribution=none  NoiseParameters=[]  Unit=N*m  AffineConversion=off  FilteringAndDerivatives=provide  SimscapeFilterOrder=1  InputFilterTimeConstant=0.001  UdotUserProvided=0
      settings: SourceProductBaseCode=SS,PW,VE
  Total Mass : fl_lib/Mechanical/Translational Elements/Mass  mass=ingenuityParams.mechanical.totalMassExceptBatteries + ingenuityParams.battery.numCells*ingenuityParams.battery.cell.mass kg  num_ports=foundation.enum.numPorts2.one  v_specify=off  v_priority=High  v=0 m/s  v_nominal_specify=off  v_nominal_unit=m/s  v_nominal_value=1  f_specify=off  f_priority=None  f=0 N  f_nominal_specify=off  f_nominal_unit=N  f_nominal_value=1
      settings: SourceProductBaseCode=PW,SS,VE  LogSimulationData=on
  T1 : PMIOPort  Side=Right
  + : PMIOPort  Port=2  Side=Left
  - : PMIOPort  Port=3  Side=Left
  T2 : PMIOPort  Port=4  Side=Right
  W : Outport
  wires:
  torRef/1 -> Simulink-PS Converter3/1
  Sensor/1 -> W/1
  PS-Simulink Converter/1 -> Sensor/1
  connections:
  Inertia1/RConn1 -- Gear Box pos/RConn1
  Inertia2/RConn1 -- Gear Box neg/RConn1
  T1/RConn1 -- Rotor1/RConn2
  Inertia1/LConn1 -- Rotor1/LConn1
  Motor & Drive/LConn1 -- +/RConn1
  Rotor1/LConn2 -- Mechanical Rotational Reference1/LConn1
  Motor & Drive/RConn2 -- PS-Simulink Converter/LConn1
  Motor & Drive/LConn2 -- Simulink-PS Converter3/RConn1
  T2/RConn1 -- Rotor2/RConn2
  Gear Box pos/LConn1 -- Motor & Drive/LConn3 -- Gear Box neg/LConn1
  Motor & Drive/RConn1 -- -/RConn1
  Motor & Drive/RConn3 -- Mechanical Rotational Reference/LConn1
  Rotor2/LConn1 -- Inertia2/LConn1
  Total Mass/LConn1 -- Rotor2/RConn1 -- Rotor1/RConn1
  Rotor2/LConn2 -- Mechanical Rotational Reference2/LConn1

== system MARS1/M.A.R.S./Force Components/Components ==
  delta : Inport
  epsilon : Inport  Port=2
  Cos : Trigonometry  Operator=cos
  Cos1 : Trigonometry  Operator=cos
  Sin : Trigonometry
  Sin1 : Trigonometry
  Out1 : Outport
  Out2 : Outport  Port=2
  Out3 : Outport  Port=3
  Out4 : Outport  Port=4
  wires:
  delta/1 -> Cos/1, Sin/1
  Sin1/1 -> Out4/1
  Cos/1 -> Out1/1
  Cos1/1 -> Out2/1
  Sin/1 -> Out3/1
  epsilon/1 -> Cos1/1, Sin1/1

== system MARS1/M.A.R.S./Force Components/Subsystem ==
  In1 : Inport
  In2 : Inport  Port=2
  In3 : Inport  Port=3
  In4 : Inport  Port=4
  In5 : Inport  Port=5
  Product : Product
  Product1 : Product
  Tcos(delta) : Product
  Tsin(delta) : Product
  Out1 : Outport
  Out2 : Outport  Port=2
  Out3 : Outport  Port=3
  wires:
  Product1/1 -> Out3/1
  In1/1 -> Tsin(delta)/1, Tcos(delta)/1
  Tsin(delta)/1 -> Product/2, Product1/1
  In4/1 -> Tsin(delta)/2
  In5/1 -> Product1/2
  Product/1 -> Out1/1
  In2/1 -> Tcos(delta)/2
  In3/1 -> Product/1
  Tcos(delta)/1 -> Out2/1

== system MARS1/Translate - Experimental/Position Hold/Distance Calc ==
  In1 : Inport
  In2 : Inport  Port=2
  Square : Math  Operator=square
  Square Root : Sqrt
  Square1 : Math  Operator=square
  Sum : Sum  Inputs=|++
  Out1 : Outport
  wires:
  Sum/1 -> Square Root/1
  Square Root/1 -> Out1/1
  Square1/1 -> Sum/2
  Square/1 -> Sum/1
  In1/1 -> Square/1
  In2/1 -> Square1/1

== system MARS1/M.A.R.S./Engine & Battery/Battery/Battery Pack ==
  Detailed Battery Pack : Subsystem  VariantControl=Detailed Battery Pack
      settings: PortSchema="{\"entries\":[{\"content\":{\"sides\":[{\"content\":{\"connectorIds\":[]},\"type\":\"ConnectorPlacement.EquallySpacedRectSide\",\"uuid\":\"ac491242-3df9-473d-beed-1a2139a6c6bd\"},{\"content\":{\"connectorIds\":[\"Out1\",\"RConn1\",\"RConn2\"],\"side\":\"RIGHT\"},\"type\":\"ConnectorPlacement.EquallySpacedRectSide\",\"uuid\":\"5d11d2aa-1dd1-475e-9911-89b4672a4360\"},{\"content\":{\"connectorIds\":[\"LConn1\"],\"side\":\"TOP\"},\"type\":\"ConnectorPlacement.EquallySpacedRectSide\",\"uuid\":\"d9fa746a-c212-49ba-8905-bd0b35a53459\"},{\"content\":{\"connectorIds\":[\"RConn3\"],\"side\":\"BOTTOM\"},\"type\":\"ConnectorPlacement.EquallySpacedRectSide\",\"uuid\":\"9203f755-4900-467a-80ce-d49a17dbef8c\"}]},\"type\":\"ConnectorPlacement.EquallySpacedConnector\",\"uuid\":\"8e24b369-26fe-4156-84c2-0f7c31bd4a1a\"}],\"packageUris\":[\"http://schema.mathworks.com/mf0/Connector/R2020b\"],\"version\":\"1.0\"}"
  Simplified Battery Pack : Subsystem  VariantControl=Simplified Battery Pack
      settings: PortSchema="{\"entries\":[{\"content\":{\"sides\":[{\"content\":{\"connectorIds\":[]},\"type\":\"ConnectorPlacement.EquallySpacedRectSide\",\"uuid\":\"ac491242-3df9-473d-beed-1a2139a6c6bd\"},{\"content\":{\"connectorIds\":[\"Out1\",\"RConn1\",\"RConn2\"],\"side\":\"RIGHT\"},\"type\":\"ConnectorPlacement.EquallySpacedRectSide\",\"uuid\":\"5d11d2aa-1dd1-475e-9911-89b4672a4360\"},{\"content\":{\"connectorIds\":[\"LConn1\"],\"side\":\"TOP\"},\"type\":\"ConnectorPlacement.EquallySpacedRectSide\",\"uuid\":\"d9fa746a-c212-49ba-8905-bd0b35a53459\"},{\"content\":{\"connectorIds\":[\"RConn3\"],\"side\":\"BOTTOM\"},\"type\":\"ConnectorPlacement.EquallySpacedRectSide\",\"uuid\":\"ceef3f59-c6c2-4ed7-8bde-a1c8d7ba1997\"}]},\"type\":\"ConnectorPlacement.EquallySpacedConnector\",\"uuid\":\"8e24b369-26fe-4156-84c2-0f7c31bd4a1a\"}],\"packageUris\":[\"http://schema.mathworks.com/mf0/Connector/R2020b\"],\"version\":\"1.0\"}"
  + : PMIOPort  Side=Left
  HEAT : PMIOPort  Port=2  Side=Right
  ENV : PMIOPort  Port=3  Side=Right
  - : PMIOPort  Port=4  Side=Right
  battery : Outport
